simulink model "test_sim"  (R2022b)
settings: Solver=ode4  StartTime=0.0  StopTime=10.0  FixedStep=0.001  RelTol=1e-3
undefined symbols (not defined in the file or in its folder): test_cal
settings Model: Creator=user  LastModifiedBy=user
settings DataIOCC: ReturnWorkspaceOutputs=off

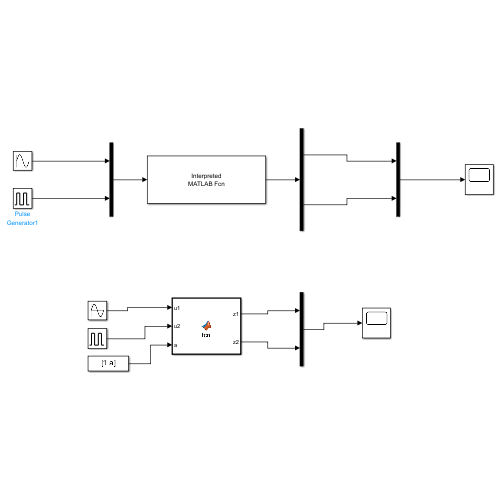
[thumbnail: Simulink's stored preview of the top-level diagram]
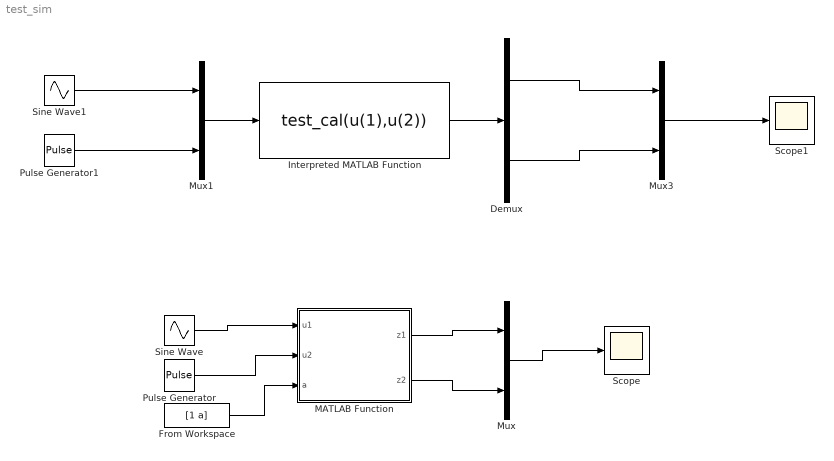
== system test_sim ==
  Demux : Demux  Outputs=2
  From Workspace : FromWorkspace  VariableName=[1 a]  SampleTime=-1  OutputAfterFinalValue=Holding final value
  Interpreted MATLAB Function : MATLABFcn  MATLABFcn=test_cal(u(1),u(2))  OutputDimensions=[2 1]  Output1D=off
  MATLAB Function : MATLAB Function  TreatAsAtomicUnit=on
  Mux : Mux  Inputs=2
  Mux1 : Mux  Inputs=2
  Mux3 : Mux  Inputs=2
  Pulse Generator : DiscretePulseGenerator  PulseType=Time based  PulseWidth=25
  Pulse Generator1 : DiscretePulseGenerator  PulseType=Time based  PulseWidth=25
  Scope : Scope
  Scope1 : Scope
  Sine Wave : Sin  SampleTime=0
  Sine Wave1 : Sin  SampleTime=0
  wires:
  Sine Wave/1 -> MATLAB Function/1(u1)
  Pulse Generator/1 -> MATLAB Function/2(u2)
  MATLAB Function/1(z1) -> Mux/1
  MATLAB Function/2(z2) -> Mux/2
  Mux/1 -> Scope/1
  From Workspace/1 -> MATLAB Function/3(a)
  Interpreted MATLAB Function/1 -> Demux/1
  Mux1/1 -> Interpreted MATLAB Function/1
  Sine Wave1/1 -> Mux1/1
  Pulse Generator1/1 -> Mux1/2
  Demux/1 -> Mux3/1
  Demux/2 -> Mux3/2
  Mux3/1 -> Scope1/1

== matlab function test_sim/MATLAB Function ==
  data: u1 input; z1 output; u2 input; z2 output; a input
function [z1,z2] = fcn(u1,u2,a)

y1 = u1 + u2;
y2 = u1 - u2;


if y1 > a
    z1 = 1;
else
    z1 = 0;
end

if y2 < -1
    z2 = -1;
else
    z2 = 0;
end
